simulink model "SPV"  (R2022b)
settings: Solver=FixedStepAuto  StartTime=0.0  StopTime=50000000  FixedStep=1  RelTol=1e-3
libraries: simulink x11
settings Model: Creator=sadamu  LastModifiedBy=程一帆
settings OptimizationCC: DefaultParameterBehavior=Inlined  DefaultUnderspecifiedDataType=single  BufferReuse=off  GlobalBufferReuse=off  ExpressionFolding=off  EnableMemcpy=off  PassReuseOutputArgsAs=Individual arguments  NoFixptDivByZeroProtection=on  EfficientFloat2IntCast=on  OptimizeDataStoreBuffers=off  BusAssignmentInplaceUpdate=off  OptimizationLevel=level0  EfficientTunableParamExpr=on
settings DebuggingCC: ParameterTunabilityLossMsg=error
settings SFSimCC: MATLABDynamicMemAlloc=off
settings RTWCC: Description=Embedded Coder  SystemTargetFile=ert.tlc  GenCodeOnly=on  TemplateMakefile=ert_default_tmf
settings CodeAppCC: GenerateComments=off  IgnoreCustomStorageClasses=off  OperatorAnnotations=on  SimulinkDataObjDesc=on  SFDataObjDesc=on  SimulinkBlockComments=off
settings ERTTargetCC: TargetLangStandard=C99 (ISO)  GenerateSampleERTMain=on  CodeInterfacePackaging=Reusable function  InlinedParameterPlacement=NonHierarchical  ERTCustomFileTemplate=example_file_process.tlc
settings ConfigComp: CovMetricSettings=dcmwe  DVMaxProcessTime=3600  DVTestSuiteOptimization=Auto  DVDetectOutOfBounds=on  DVModelReferenceHarness=on

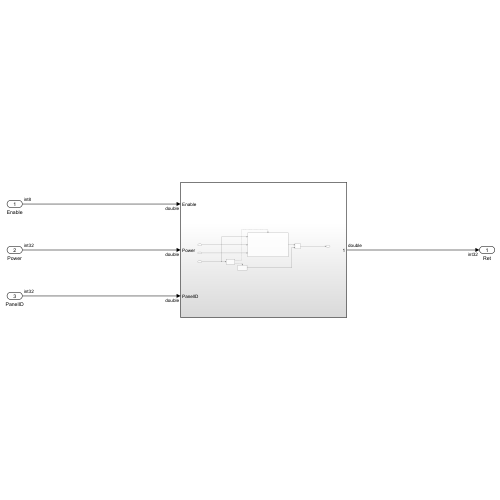
[thumbnail: Simulink's stored preview of the top-level diagram]
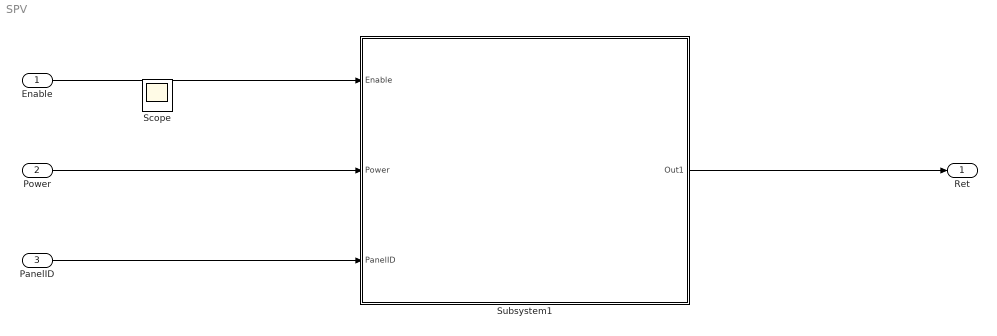
== system SPV ==
  Enable : Inport  OutDataTypeStr=int8
  Power : Inport  Port=2  OutDataTypeStr=int32
  PanelID : Inport  Port=3  OutDataTypeStr=int32
  Subsystem1 : Subsystem
  Ret : Outport
  Scope : Scope
  wires:
  Enable/1 -> Subsystem1/1(Enable)
  Power/1 -> Subsystem1/2(Power)
  PanelID/1 -> Subsystem1/3(PanelID)
  Subsystem1/1(Out1) -> Ret/1

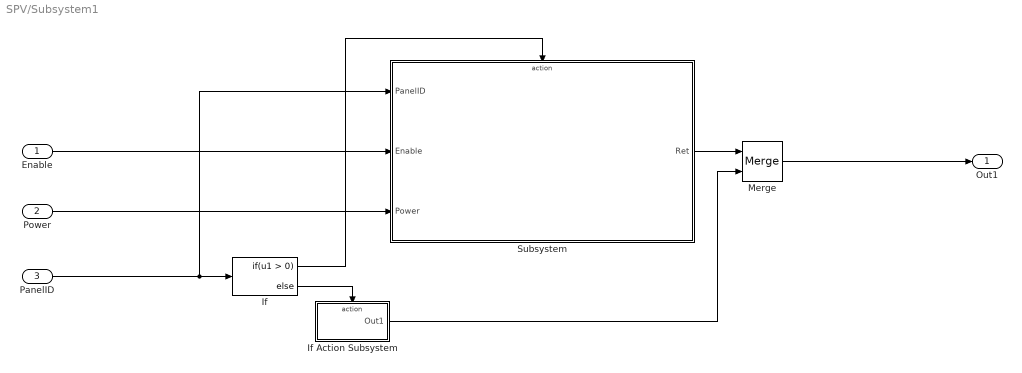
== system SPV/Subsystem1 ==
  Enable : Inport
  Power : Inport  Port=2
  PanelID : Inport  Port=3
  If : If
  If Action Subsystem : Subsystem  TreatAsAtomicUnit=on
  Merge : Merge
  Subsystem : Subsystem  mask{Len=16}
      mask DialogControl ParameterGroupVar Prompt: 参数
  Out1 : Outport
  wires:
  If Action Subsystem/1(Out1) -> Merge/2
  If/1 -> Subsystem/Action
  PanelID/1 -> Subsystem/1(PanelID), If/1
  Merge/1 -> Out1/1
  If/2 -> If Action Subsystem/Action
  Power/1 -> Subsystem/3(Power)
  Subsystem/1(Ret) -> Merge/1
  Enable/1 -> Subsystem/2(Enable)

== system SPV/Subsystem1/If Action Subsystem ==
  Action Port : ActionPort  ActionPortLabel=else
  Constant : Constant  Value=-1  OutDataTypeStr=int32
  Out1 : Outport
  wires:
  Constant/1 -> Out1/1

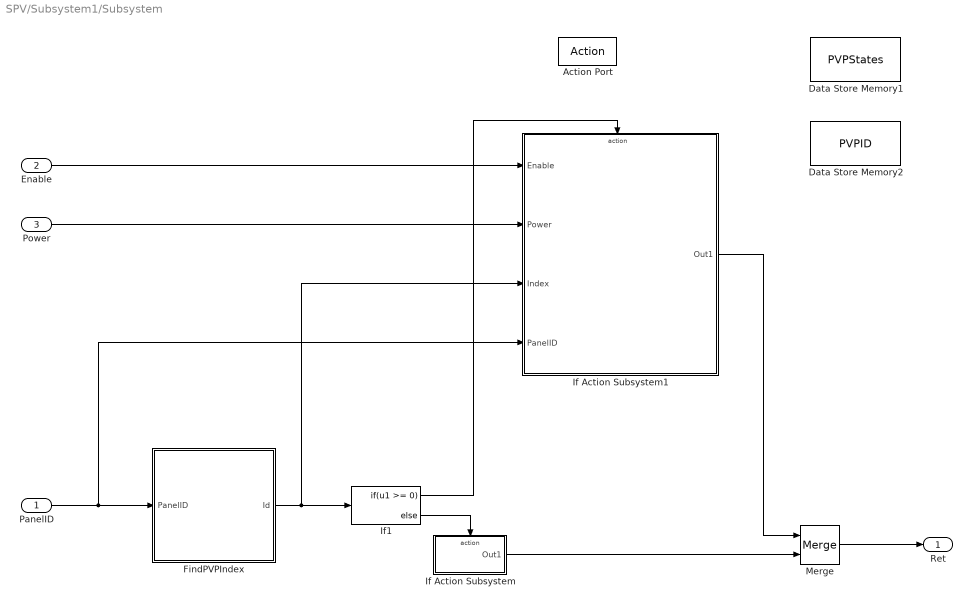
== system SPV/Subsystem1/Subsystem ==
  PanelID : Inport  OutDataTypeStr=int32
  Enable : Inport  Port=2
  Power : Inport  Port=3
  Action Port : ActionPort  ActionPortLabel=if(u1 > 0)
  Data Store Memory1 : DataStoreMemory  DataStoreName=PVPStates  WriteAfterWriteMsg=warning  ShowAdditionalParam=off  OutDataTypeStr=int32  Dimensions=Len
  Data Store Memory2 : DataStoreMemory  DataStoreName=PVPID  WriteAfterWriteMsg=warning  ShowAdditionalParam=off  OutDataTypeStr=int32  Dimensions=Len
  FindPVPIndex : Subsystem  TreatAsAtomicUnit=on
  If Action Subsystem : Subsystem  TreatAsAtomicUnit=on
  If Action Subsystem1 : Subsystem  TreatAsAtomicUnit=on
  If1 : If  IfExpression=u1 >= 0
  Merge : Merge
  Ret : Outport
  wires:
  Merge/1 -> Ret/1
  If1/1 -> If Action Subsystem1/Action
  Power/1 -> If Action Subsystem1/2(Power)
  If1/2 -> If Action Subsystem/Action
  FindPVPIndex/1(Id) -> If Action Subsystem1/3(Index), If1/1
  Enable/1 -> If Action Subsystem1/1(Enable)
  If Action Subsystem/1(Out1) -> Merge/2
  If Action Subsystem1/1(Out1) -> Merge/1
  PanelID/1 -> If Action Subsystem1/4(PanelID), FindPVPIndex/1(PanelID)

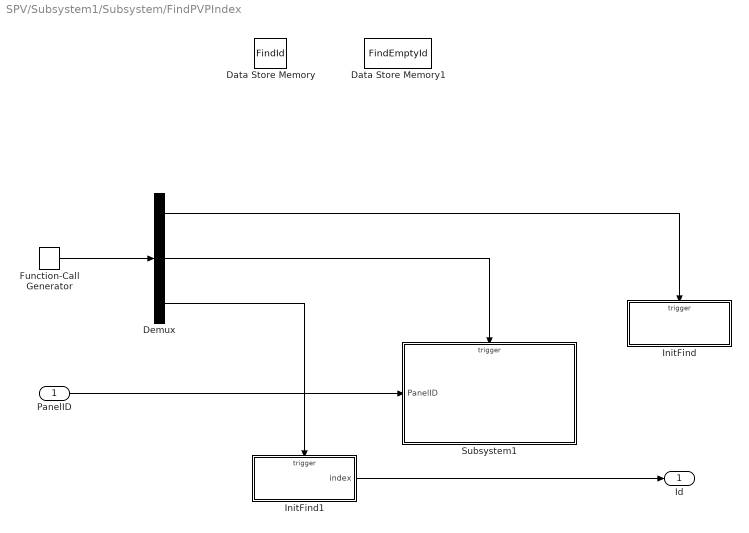
== system SPV/Subsystem1/Subsystem/FindPVPIndex ==
  PanelID : Inport
  Data Store Memory : DataStoreMemory  DataStoreName=FindId  WriteAfterWriteMsg=warning  ShowAdditionalParam=off  OutDataTypeStr=int32
  Data Store Memory1 : DataStoreMemory  DataStoreName=FindEmptyId  WriteAfterWriteMsg=warning  ShowAdditionalParam=off  OutDataTypeStr=int32
  Demux : Demux  Outputs=3
  Function-Call Generator : simulink/Ports & Subsystems/Function-Call Generator  sample_time=1  numberOfIterations=1  DisallowWideOutput=off
  InitFind : Subsystem
  InitFind1 : Subsystem
  Subsystem1 : Subsystem
  Id : Outport
  wires:
  Function-Call Generator/1 -> Demux/1
  Demux/1 -> InitFind/Trigger
  Demux/2 -> Subsystem1/Trigger
  PanelID/1 -> Subsystem1/1(PanelID)
  InitFind1/1(index) -> Id/1
  Demux/3 -> InitFind1/Trigger

== system SPV/Subsystem1/Subsystem/If Action Subsystem ==
  Action Port : ActionPort  ActionPortLabel=else
  Constant : Constant  Value=-2  OutDataTypeStr=int32
  Out1 : Outport
  wires:
  Constant/1 -> Out1/1

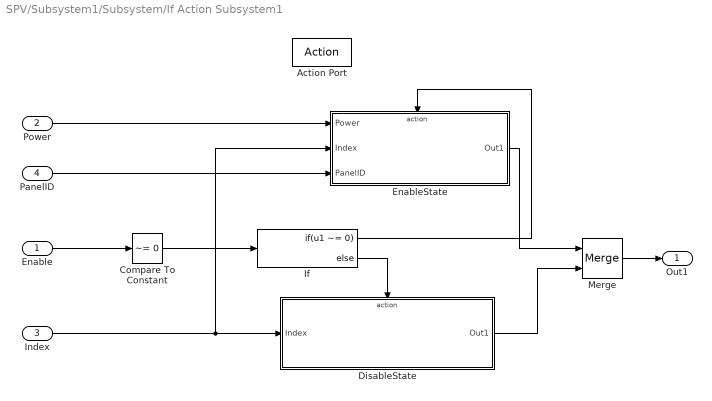
== system SPV/Subsystem1/Subsystem/If Action Subsystem1 ==
  Enable : Inport
  Power : Inport  Port=2
  Index : Inport  Port=3  OutDataTypeStr=int32
  PanelID : Inport  Port=4
  Action Port : ActionPort  ActionPortLabel=if(u1 >= 0)
  Compare To Constant : simulink/Logic and Bit Operations/Compare To Constant  relop=~=  const=0  OutDataTypeStr=boolean
  DisableState : Subsystem  TreatAsAtomicUnit=on
  EnableState : Subsystem  TreatAsAtomicUnit=on
  If : If  IfExpression=u1 ~= 0
  Merge : Merge
  Out1 : Outport
  wires:
  EnableState/1(Out1) -> Merge/1
  Power/1 -> EnableState/1(Power)
  Index/1 -> EnableState/2(Index), DisableState/1(Index)
  Compare To Constant/1 -> If/1
  If/2 -> DisableState/Action
  Enable/1 -> Compare To Constant/1
  If/1 -> EnableState/Action
  PanelID/1 -> EnableState/3(PanelID)
  DisableState/1(Out1) -> Merge/2
  Merge/1 -> Out1/1

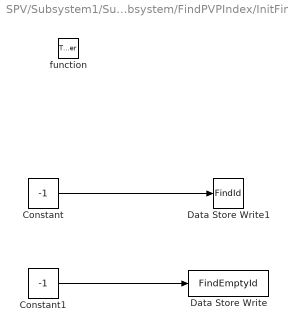
== system SPV/Subsystem1/Subsystem/FindPVPIndex/InitFind ==
  function : TriggerPort  TriggerType=function-call  VariantControl=Variant
  Constant : Constant  Value=-1  OutDataTypeStr=int32
  Constant1 : Constant  Value=-1  OutDataTypeStr=int32
  Data Store Write : DataStoreWrite  DataStoreName=FindEmptyId  IndexOptions=Index vector (dialog)  Indices=1  OutputSizes=1
  Data Store Write1 : DataStoreWrite  DataStoreName=FindId  IndexOptions=Index vector (dialog)  Indices=1  OutputSizes=1
  wires:
  Constant/1 -> Data Store Write1/1
  Constant1/1 -> Data Store Write/1

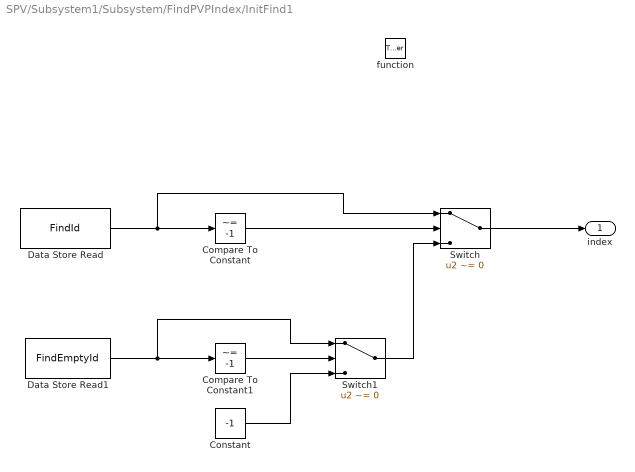
== system SPV/Subsystem1/Subsystem/FindPVPIndex/InitFind1 ==
  function : TriggerPort  TriggerType=function-call  VariantControl=Variant
  Compare To Constant : simulink/Logic and Bit Operations/Compare To Constant  relop=~=  const=-1  OutDataTypeStr=boolean
  Compare To Constant1 : simulink/Logic and Bit Operations/Compare To Constant  relop=~=  const=-1  OutDataTypeStr=boolean
  Constant : Constant  Value=-1  OutDataTypeStr=int16
  Data Store Read : DataStoreRead  DataStoreName=FindId  IndexOptions=Index vector (dialog)  Indices=1  OutputSizes=1
  Data Store Read1 : DataStoreRead  DataStoreName=FindEmptyId  IndexOptions=Index vector (dialog)  Indices=1  OutputSizes=1
  Switch : Switch  Criteria=u2 ~= 0  SaturateOnIntegerOverflow=off  InputSameDT=off
  Switch1 : Switch  Criteria=u2 ~= 0  SaturateOnIntegerOverflow=off  InputSameDT=off
  index : Outport
  wires:
  Data Store Read/1 -> Switch/1, Compare To Constant/1
  Compare To Constant/1 -> Switch/2
  Data Store Read1/1 -> Switch1/1, Compare To Constant1/1
  Compare To Constant1/1 -> Switch1/2
  Switch1/1 -> Switch/3
  Constant/1 -> Switch1/3
  Switch/1 -> index/1

== system SPV/Subsystem1/Subsystem/FindPVPIndex/Subsystem1 ==
  PanelID : Inport
  function : TriggerPort  TriggerType=function-call  VariantControl=Variant
  Subsystem : Subsystem
  wires:
  PanelID/1 -> Subsystem/1(PanelID)

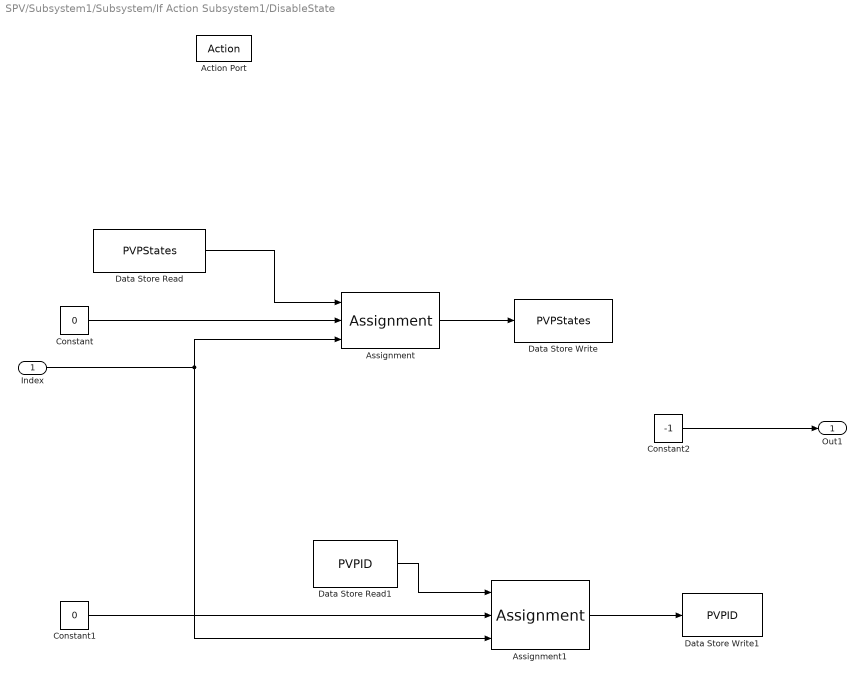
== system SPV/Subsystem1/Subsystem/If Action Subsystem1/DisableState ==
  Index : Inport
  Action Port : ActionPort  ActionPortLabel=else
  Assignment : Assignment  IndexMode=Zero-based  DiagnosticForDimensions=Warning  IndexOptions=Index vector (port)  Indices=1  OutputSizes=1
  Assignment1 : Assignment  IndexMode=Zero-based  DiagnosticForDimensions=Warning  IndexOptions=Index vector (port)  Indices=1  OutputSizes=1
  Constant : Constant  Value=0  OutDataTypeStr=int32
  Constant1 : Constant  Value=0  OutDataTypeStr=int32
  Constant2 : Constant  Value=-1  OutDataTypeStr=int32
  Data Store Read : DataStoreRead  DataStoreName=PVPStates  IndexOptions=Index vector (dialog)  Indices=1  OutputSizes=1
  Data Store Read1 : DataStoreRead  DataStoreName=PVPID  IndexOptions=Index vector (dialog)  Indices=1  OutputSizes=1
  Data Store Write : DataStoreWrite  DataStoreName=PVPStates  IndexOptions=Index vector (dialog)  Indices=1  OutputSizes=1
  Data Store Write1 : DataStoreWrite  DataStoreName=PVPID  IndexOptions=Index vector (dialog)  Indices=1  OutputSizes=1
  Out1 : Outport
  wires:
  Data Store Read/1 -> Assignment/1
  Assignment/1 -> Data Store Write/1
  Data Store Read1/1 -> Assignment1/1
  Index/1 -> Assignment1/3, Assignment/3
  Assignment1/1 -> Data Store Write1/1
  Constant/1 -> Assignment/2
  Constant1/1 -> Assignment1/2
  Constant2/1 -> Out1/1

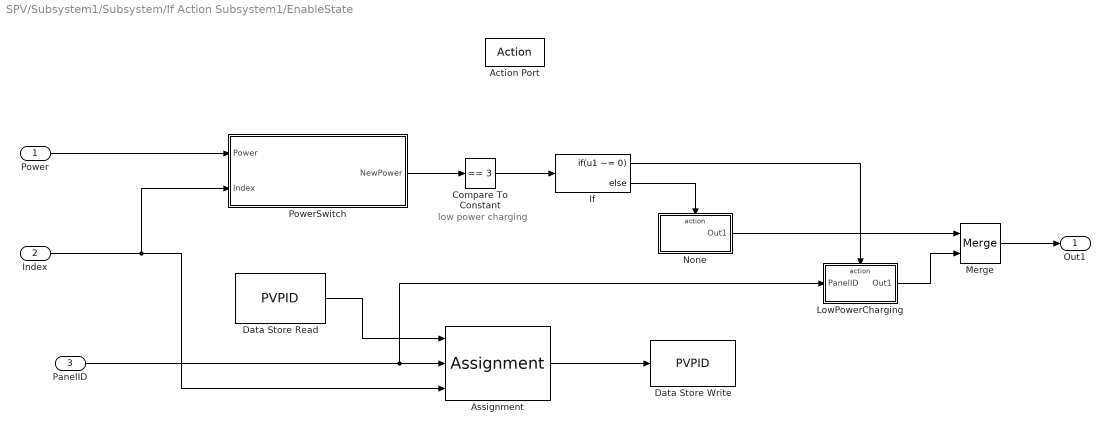
== system SPV/Subsystem1/Subsystem/If Action Subsystem1/EnableState ==
  note: low power charging
  Power : Inport
  Index : Inport  Port=2  OutDataTypeStr=int32
  PanelID : Inport  Port=3
  Action Port : ActionPort  ActionPortLabel=if(u1 ~= 0)
  Assignment : Assignment  IndexMode=Zero-based  DiagnosticForDimensions=Warning  IndexOptions=Index vector (port)  Indices=1  OutputSizes=1
  Compare To Constant : simulink/Logic and Bit Operations/Compare To Constant  relop===  const=3  OutDataTypeStr=boolean
  Data Store Read : DataStoreRead  DataStoreName=PVPID  IndexOptions=Index vector (dialog)  Indices=1  OutputSizes=1
  Data Store Write : DataStoreWrite  DataStoreName=PVPID  IndexOptions=Index vector (dialog)  Indices=1  OutputSizes=1
  If : If  IfExpression=u1 ~= 0
  LowPowerCharging : Subsystem  TreatAsAtomicUnit=on
  Merge : Merge
  None : Subsystem  TreatAsAtomicUnit=on
  PowerSwitch : Subsystem  TreatAsAtomicUnit=on
  Out1 : Outport
  wires:
  Power/1 -> PowerSwitch/1(Power)
  Index/1 -> Assignment/3, PowerSwitch/2(Index)
  Assignment/1 -> Data Store Write/1
  Data Store Read/1 -> Assignment/1
  PanelID/1 -> LowPowerCharging/1(PanelID), Assignment/2
  PowerSwitch/1(NewPower) -> Compare To Constant/1
  Compare To Constant/1 -> If/1
  If/1 -> LowPowerCharging/Action
  If/2 -> None/Action
  None/1(Out1) -> Merge/1
  LowPowerCharging/1(Out1) -> Merge/2
  Merge/1 -> Out1/1

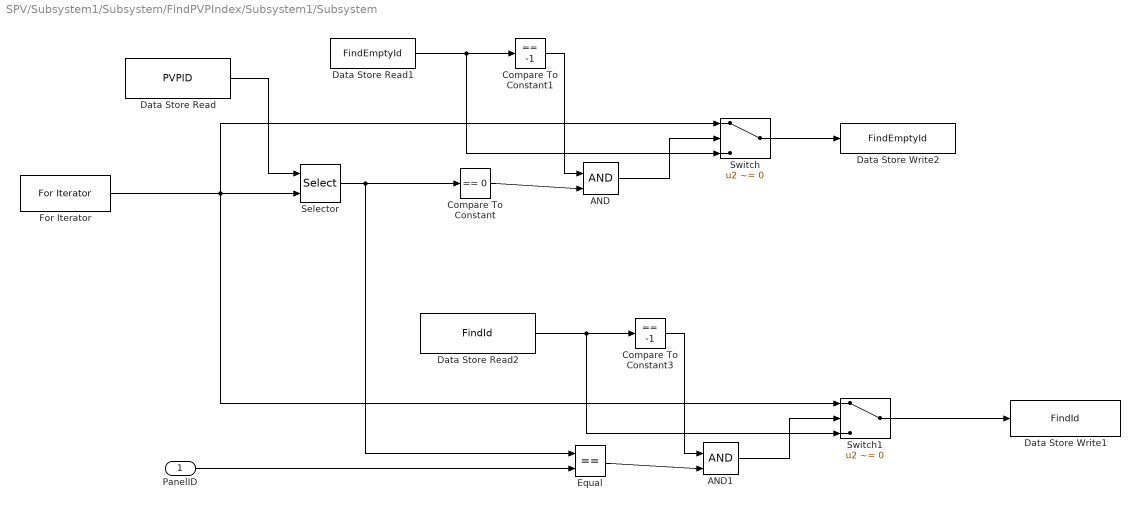
== system SPV/Subsystem1/Subsystem/FindPVPIndex/Subsystem1/Subsystem ==
  PanelID : Inport
  AND : Logic  IconShape=distinctive  AllPortsSameDT=off  OutDataTypeStr=boolean
  AND1 : Logic  IconShape=distinctive  AllPortsSameDT=off  OutDataTypeStr=boolean
  Compare To Constant : simulink/Logic and Bit Operations/Compare To Constant  relop===  const=0  OutDataTypeStr=boolean
  Compare To Constant1 : simulink/Logic and Bit Operations/Compare To Constant  relop===  const=-1  OutDataTypeStr=boolean
  Compare To Constant3 : simulink/Logic and Bit Operations/Compare To Constant  relop===  const=-1  OutDataTypeStr=boolean
  Data Store Read : DataStoreRead  DataStoreName=PVPID  IndexOptions=Index vector (dialog)  Indices=1  OutputSizes=1
  Data Store Read1 : DataStoreRead  DataStoreName=FindEmptyId  IndexOptions=Index vector (dialog)  Indices=1  OutputSizes=1
  Data Store Read2 : DataStoreRead  DataStoreName=FindId  IndexOptions=Index vector (dialog)  Indices=1  OutputSizes=1
  Data Store Write1 : DataStoreWrite  DataStoreName=FindId  IndexOptions=Index vector (dialog)  Indices=1  OutputSizes=1
  Data Store Write2 : DataStoreWrite  DataStoreName=FindEmptyId  IndexOptions=Index vector (dialog)  Indices=1  OutputSizes=1
  Equal : RelationalOperator  Operator===  OutDataTypeStr=boolean  RndMeth=Simplest  InputSameDT=off
  For Iterator : ForIterator  IterationLimit=Len  IndexMode=Zero-based
  Selector : Selector  IndexMode=Zero-based  InputPortWidth=Len  IndexOptions=Index vector (port)  Indices=[1 3]  OutputSizes=1
  Switch : Switch  Criteria=u2 ~= 0  SaturateOnIntegerOverflow=off  InputSameDT=off
  Switch1 : Switch  Criteria=u2 ~= 0  SaturateOnIntegerOverflow=off  InputSameDT=off
  wires:
  Data Store Read/1 -> Selector/1
  Selector/1 -> Equal/1, Compare To Constant/1
  Compare To Constant/1 -> AND/2
  Data Store Read1/1 -> Switch/3, Compare To Constant1/1
  Compare To Constant1/1 -> AND/1
  AND/1 -> Switch/2
  Switch/1 -> Data Store Write2/1
  Equal/1 -> AND1/2
  AND1/1 -> Switch1/2
  Compare To Constant3/1 -> AND1/1
  Data Store Read2/1 -> Switch1/3, Compare To Constant3/1
  Switch1/1 -> Data Store Write1/1
  PanelID/1 -> Equal/2
  For Iterator/1 -> Switch1/1, Switch/1, Selector/2

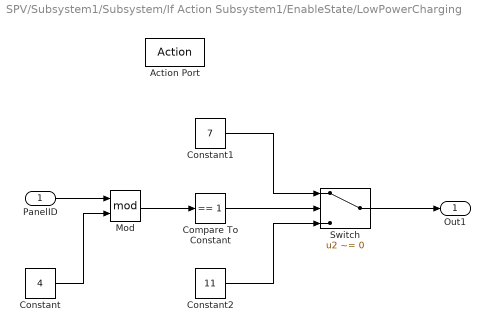
== system SPV/Subsystem1/Subsystem/If Action Subsystem1/EnableState/LowPowerCharging ==
  PanelID : Inport
  Action Port : ActionPort  ActionPortLabel=if(u1 ~= 0)
  Compare To Constant : simulink/Logic and Bit Operations/Compare To Constant  relop===  const=1  OutDataTypeStr=boolean
  Constant : Constant  Value=4  OutDataTypeStr=int32
  Constant1 : Constant  Value=7  OutDataTypeStr=int32
  Constant2 : Constant  Value=11  OutDataTypeStr=int32
  Mod : Math  Operator=mod
  Switch : Switch  Criteria=u2 ~= 0  SaturateOnIntegerOverflow=off  InputSameDT=off
  Out1 : Outport
  wires:
  Constant/1 -> Mod/2
  PanelID/1 -> Mod/1
  Mod/1 -> Compare To Constant/1
  Compare To Constant/1 -> Switch/2
  Constant1/1 -> Switch/1
  Constant2/1 -> Switch/3
  Switch/1 -> Out1/1

== system SPV/Subsystem1/Subsystem/If Action Subsystem1/EnableState/None ==
  Action Port : ActionPort  ActionPortLabel=else
  Constant : Constant  OutDataTypeStr=int32
  Out1 : Outport
  wires:
  Constant/1 -> Out1/1

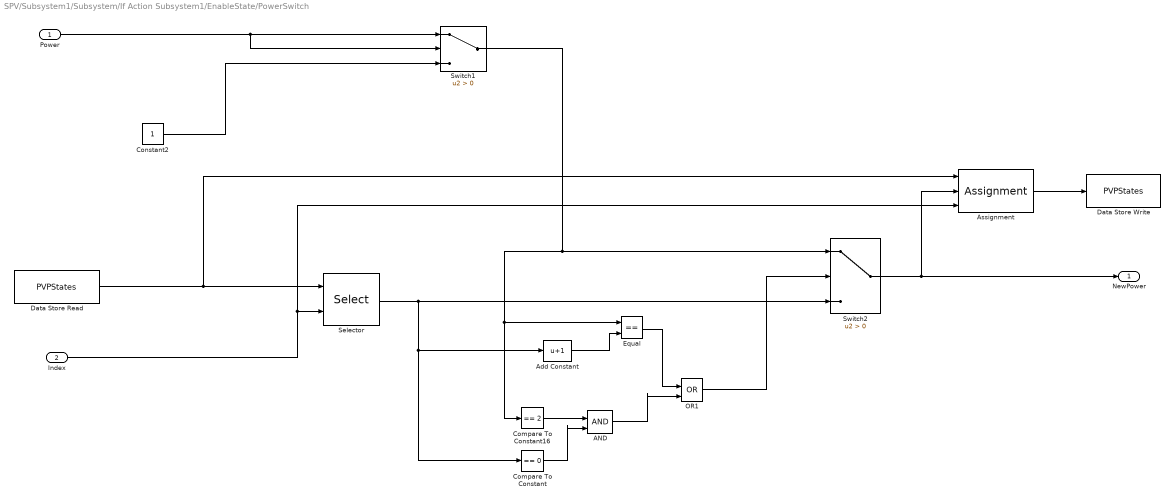
== system SPV/Subsystem1/Subsystem/If Action Subsystem1/EnableState/PowerSwitch ==
  Power : Inport
  Index : Inport  Port=2  OutDataTypeStr=int32
  AND : Logic  IconShape=distinctive  AllPortsSameDT=off  OutDataTypeStr=boolean
  Add Constant : Bias  Bias=1  SaturateOnIntegerOverflow=off
  Assignment : Assignment  IndexMode=Zero-based  DiagnosticForDimensions=Warning  IndexOptions=Index vector (port)  Indices=1  OutputSizes=1
  Compare To Constant : simulink/Logic and Bit Operations/Compare To Constant  relop===  const=0  OutDataTypeStr=boolean
  Compare To Constant16 : simulink/Logic and Bit Operations/Compare To Constant  relop===  const=2  OutDataTypeStr=boolean
  Constant2 : Constant  OutDataTypeStr=int32
  Data Store Read : DataStoreRead  DataStoreName=PVPStates  IndexOptions=Index vector (dialog)  Indices=1  OutputSizes=1
  Data Store Write : DataStoreWrite  DataStoreName=PVPStates  IndexOptions=Index vector (dialog)  Indices=1  OutputSizes=1
  Equal : RelationalOperator  Operator===  OutDataTypeStr=boolean  RndMeth=Simplest  InputSameDT=off
  OR1 : Logic  Operator=OR  IconShape=distinctive  AllPortsSameDT=off  OutDataTypeStr=boolean
  Selector : Selector  IndexMode=Zero-based  InputPortWidth=Len  IndexOptions=Index vector (port)  Indices=[1 3]  OutputSizes=1
  Switch1 : Switch  Criteria=u2 > Threshold  SaturateOnIntegerOverflow=off  InputSameDT=off
  Switch2 : Switch  Criteria=u2 > Threshold  SaturateOnIntegerOverflow=off  InputSameDT=off
  NewPower : Outport
  wires:
  Switch1/1 -> Compare To Constant16/1, Equal/1, Switch2/1
  Data Store Read/1 -> Assignment/1, Selector/1
  Constant2/1 -> Switch1/3
  Assignment/1 -> Data Store Write/1
  Index/1 -> Assignment/3, Selector/2
  OR1/1 -> Switch2/2
  Selector/1 -> Add Constant/1, Compare To Constant/1, Switch2/3
  Switch2/1 -> NewPower/1, Assignment/2
  Power/1 -> Switch1/2, Switch1/1
  Compare To Constant16/1 -> AND/1
  Compare To Constant/1 -> AND/2
  Add Constant/1 -> Equal/2
  Equal/1 -> OR1/1
  AND/1 -> OR1/2
